simulink model "sim_switc_hover_vol_rotation"  (R2020b)
settings: Solver=VariableStepAuto  StartTime=0.0  StopTime=T  MaxStep=MaxStep  RelTol=RelTol
values from neighbouring files (symbols this model uses):
  a = 400    [switch_hovering_vol_rotation.m]
  b = 500    [switch_hovering_vol_rotation.m]
  controlleur = generateContolleur(drone)    [switch_hovering_vol_rotation.m]
  drone = generateDarko()    [switch_hovering_vol_rotation.m]
  J = 200    [switch_hovering_vol_rotation.m]
  K_complet = [K(:,1:6), [0;0;0;0], K(:,7:12)]    [switch_hovering_vol_rotation.m]
  rule = 1    [switch_hovering_vol_rotation.m]
  S_complet = [S(1:6,1:6), zeros(6,1), S(1:6,7:12); zeros(1,13); S(7:12,1:6), zeros(6,1), S(7:12,7:12)]    [switch_hovering_vol_rotation.m]
  T = 80    [switch_hovering_vol_rotation.m]
  u_eq_hover = drone.G*drone.MASS/(2*drone.Fb(1,1)) * [1;1;0;0]    [switch_hovering_vol_rotation.m]
  x0 = [p_initial; v_initial; q_initial; omega_initial; s]    [switch_hovering_vol_rotation.m]
  x_eq_hover = [[0; 0; 0]; [0; 0; 0]; [1/sqrt(2); 0; -1/sqrt(2);0]; [0; 0; 0]]    [switch_hovering_vol_rotation.m]
undefined symbols (not defined in the file or in its folder): f_initial, q_d_initial, speed
libraries: simulink_extras x5, simulink x3, pid_lib x1, sharedtransform x1
(part 2 of 2)

== matlab function sim_switc_hover_vol_rotation/Controlleur_vol_NL/Subsystem/distri ==
  data: x input; T1pT2 input; tau input; u_barre input; u_barre_dot output; controlleur parameter; drone parameter; conv output; W output; determinant output; s output; M output
function [u_barre_dot, conv,W, determinant, s, M]= dist(x, T1pT2, tau, u_barre, controlleur, drone)

% p = x(1:3);
v = x(4:6);
q  = x(7:10);
w = x(11:13);

T1mT2 = u_barre(1);
d1pd2 = u_barre(2);
d1md2 = u_barre(3);


D = q2dcm(q);

%% velocityin body frame
vb = D'*v;
vbx = vb(1);
vby = vb(2);
vbz = vb(3);

J = drone.INERTIA;


ay = drone.P_A2_CG(2);
py = drone.P_P2_CG(2);
die_c = drone.PHI(3,3);
Cd0 = drone.PHI(1,1);

Swet   = drone.WET_SURFACE;
Sdry   = drone.DRY_SURFACE;
Sp = pi*drone.PROP_RADIUS^2;
Thetam = drone.ELEVON_MEFFICIENCY(2);
Thetaf = drone.ELEVON_FEFFICIENCY(2);
kf = drone.PROP_KP;
km = drone.PROP_KM;
S = Swet + Sdry;
rho    = drone.RHO;
phi_n  = drone.PHI_n;
chord  = drone.CHORD;
ws     = drone.WINGSPAN;
B = diag([ws; chord; ws]);
dR = drone.CENTRAGE ;

eta = sqrt( norm(v)^2 + phi_n*norm(B*w)^2 );

% M = [
% (km/kf - (Swet/(8*Sp)) * ay * die_c * Thetaf *d1pd2)*T1mT2 + (-(Swet/(8*Sp))* ay * die_c * Thetaf* T1pT2 + 1/4 * rho* S * eta * ay * die_c * Thetaf* vbx)*d1md2; 
% (Swet/(8*Sp) * dR * die_c * Thetam * T1pT2 + 1/4 * rho* S * eta * dR * die_c * Thetam* vbx )* d1pd2 + Swet/(8*Sp) * dR * die_c * Thetam * T1mT2*d1md2 + 1/2 * rho* S *  dR  * die_c * eta *vbz ;
% -(py+Swet/(4*Sp)*ay*Cd0)*T1mT2 + (1/4 * rho* S * eta * ay * Cd0 * Thetaf* vbz)*d1md2
%     ];

x= T1mT2 ;
y = d1pd2;
z = d1md2;

M = [
(km/kf - (Swet/(8*Sp)) * ay * die_c * Thetaf *y)*x + (-(Swet/(8*Sp))* ay * die_c * Thetaf* T1pT2 + 1/4 * rho* S * eta * ay * die_c * Thetaf* vbx)*z; 
(Swet/(8*Sp) * dR * die_c * Thetam * T1pT2 + 1/4 * rho* S * eta * dR * die_c * Thetam* vbx )* y + Swet/(8*Sp) * dR * die_c * Thetam * x*z + 1/2 * rho* S *  dR  * die_c * eta *vbz ;
-(py+Swet/(4*Sp)*ay*Cd0)*x + (1/4 * rho* S * eta * ay * Cd0 * Thetaf* vbz)*z
    ];

% M =J*M;
 
dM = [km/kf - (Swet/(8*Sp)) * ay * die_c * Thetaf *d1pd2, -(Swet/(8*Sp))* ay * die_c * Thetaf * T1mT2 ,(-(Swet/(8*Sp))* ay * die_c * Thetaf* T1pT2 + 1/4 * rho* S * eta * ay * die_c * Thetaf* vbx);
(Swet/(8*Sp) * dR * die_c * Thetam * d1md2), Swet/(8*Sp) * dR * die_c * Thetam * T1pT2 + 1/4 * rho* S * eta * dR * die_c * Thetam* vbx, Swet/(8*Sp) * dR * die_c * Thetam * T1mT2;
-(py+Swet/(4*Sp)*ay*Cd0), 0, 1/4 * rho* S * eta * ay * Cd0 * Thetaf* vbz
     ];
% dM = J*dM;

sat_val = 10000;
[U,S,V] = svd(dM);

inv_S = zeros(3);
inv_S(1,1) = min(sat_val, max(-sat_val, 1/S(1,1)));
inv_S(2,2) = min(sat_val, max(-sat_val, 1/S(2,2)));
inv_S(3,3) = min(sat_val, max(-sat_val, 1/S(3,3)));

% inv_dM = V*inv(S)*U';
inv_dM = V*inv_S*U';

% u_barre_dot = - controlleur.ku * inv(dM)*(M - tau );
u_barre_dot = - controlleur.ku * inv_dM*(M - tau );

conv= M - tau ;
W = (M - tau)'*(M - tau);
determinant = det(dM);
s = dM*u_barre_dot;

== matlab function sim_switc_hover_vol_rotation/Controlleur_vol_NL/vecteur de commande ==
  data: cmd_vect input; u output
function u = fcn(cmd_vect)

T1pT2 = cmd_vect(1);
T1mT2 = cmd_vect(2);
d1pd2 = cmd_vect(3);
d1md2 = cmd_vect(4);

u = [1/2*(T1pT2 + T1mT2); 1/2*(T1pT2 - T1mT2); 1/2*(d1pd2 + d1md2); 1/2*(d1pd2 - d1md2)];

== matlab function sim_switc_hover_vol_rotation/Controlleur_vol_NL/Adaptation ==
  data: u input; u_adapt output
function u_adapt = fcn(u)

T1 = u(1);
T2 = u(2);
d1 = u(3);
d2 = u(4);

u_adapt = [T1; T2; T1*d1; T2*d2];

== matlab function sim_switc_hover_vol_rotation/Controlleur_hover_NL_rot/dem ==
  data: x input; p_v output; q_omega output
function [p_v, q_omega] = demux(x)

p_v = x(1:6);
q_omega = x(7:13);

== matlab function sim_switc_hover_vol_rotation/Controlleur_hover_NL_rot/stabilizer_q_omega ==
  data: q_d input; omega_d input; omega_dd input; q_omega input; tau_r output; controlleur parameter; drone parameter; q_delta output; omega_delta output
function [tau_r, q_delta, omega_delta]  = stabilizer_q_omega(q_d, omega_d, omega_dd, q_omega, controlleur, drone )

J = drone.INERTIA;

q = q_omega(1:4);
omega = q_omega(5:7);

eta = q(1);
eps = q(2:4);

eta_d = q_d(1);
eps_d = q_d(2:4);

eta_delta = eta_d*eta + eps_d'*eps;
eps_delta = -eta*eps_d + eta_d*eps - skew_sym(eps_d)*eps;

omega_delta = omega - omega_d;

tau_r = - controlleur.kap * eps_delta - controlleur.kad * omega_delta + cross(omega, J* omega) + J*omega_dd;
q_delta = [eta_delta; eps_delta];
end

== matlab function sim_switc_hover_vol_rotation/Controlleur_hover_NL_rot/split ==
  data: f input; nu input; f_d output size=1; q_d input; q_r input; omega_d output size=3; controlleur parameter; err output
function [f_d, omega_d, err] = split(f, nu, q_d, q_r, controlleur)
%#codegen

R_d = q2dcm(q_d);

eta_d = q_d(1);
eps_d = q_d(2:4);

eta_r = q_r(1);
eps_r = q_r(2:4);

eps_delta_prime = -eta_d*eps_r + eta_r*eps_d - skew_sym(eps_r)*eps_d;

f_d = (R_d * controlleur.d_etoile)' * nu;
omega_d = 1/f * controlleur.skew_sym_d_etoile * R_d' * nu -controlleur.kq*controlleur.d_etoile*controlleur.d_etoile'*eps_delta_prime;

err =  R_d*controlleur.d_etoile*f_d + skew_sym(omega_d) * controlleur.d_etoile * f - nu;

== matlab function sim_switc_hover_vol_rotation/Controlleur_hover_NL_rot/f_delta stab ==
  data: f input; f_delta input; nu output; e input; q_omega input; q_d input; controlleur parameter; drone parameter
function nu = stab_f_delta(f, f_delta, e, q_omega, q_d, controlleur, drone)
%#codegen
m = drone.MASS;
kpp = controlleur.kpp;
kpd = controlleur.kpd;
k_delta = controlleur.k_delta;

ep = e(1:3);
ev = e(4:6);

q = q_omega(1:4);
% omega = q_omega(5:7);

R = q2dcm(q);
Rd = q2dcm(q_d);

nu = ((kpp * kpd)/m) * ep + (kpd^2/m - kpp) * ev - (kpd/m + k_delta) * f_delta -kpd/m * (R-Rd) * controlleur.d_etoile * f;

== matlab function sim_switc_hover_vol_rotation/MATLAB Function3 ==
  data: u input; y output
function y = fcn(u)
%#codegen

y = norm(u);

== matlab function sim_switc_hover_vol_rotation/Controlleur_hover_NL_rot/e stab ==
  data: e input; f_r output; drone parameter; controlleur parameter
function f_r = e_stab(e, drone, controlleur)
%#codegen
ep = e(1:3);
ev = e(4:6);

f_r = drone.MASS * [0;0;drone.G] - controlleur.kpp * ep - controlleur.kpd * ev;
